simulink model "shape_delay_atten_noComp"  (R2022a)
settings: Solver=FixedStepAuto  StartTime=0.0  StopTime=10.0  RelTol=1e-3
values from neighbouring files (symbols this model uses):
  f_atten = 0.1    [zz_noShape.m]
  scale_LED = a_LED(numel(a_LED)) * A0_stage^num_LED    [zz_noShape.m]
  scale_ZCD = a_ZCD(numel(a_ZCD)) * A0_stage^num_ZCD    [zz_noShape.m]
  t_delay = shaper_struct.t_delay;'    [sim_shaper.m]    (also in zz_cfd.m = 2e-9;'; zz_noShape.m = 1.337e-08)
  v_threshold = (1.8/(2^9)) * 71    (= 0.249609375)    [zz_noShape.m]
  voff_led = 0.0    (= 0)    [zz_noShape.m]
  voff_zcd = 0.0    (= 0)    [zz_noShape.m]
undefined symbols (not defined in the file or in its folder): a_LED, a_ZCD, b_LED, b_ZCD
settings Model: Creator=lydialee  LastModifiedBy=lydialee
settings SolverCC: MaxZcPerStep=1
settings DataIOCC: ExternalInput=[t_vec, v_in]

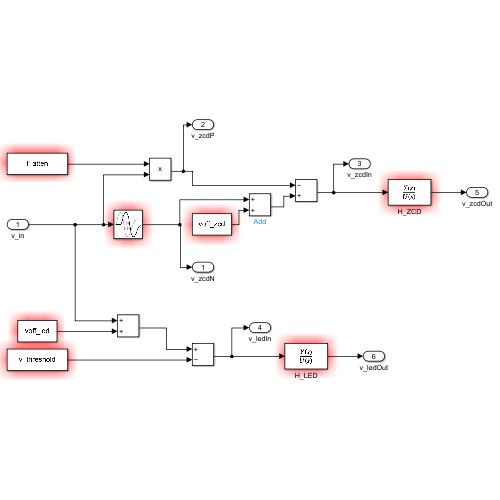
[thumbnail: Simulink's stored preview of the top-level diagram]
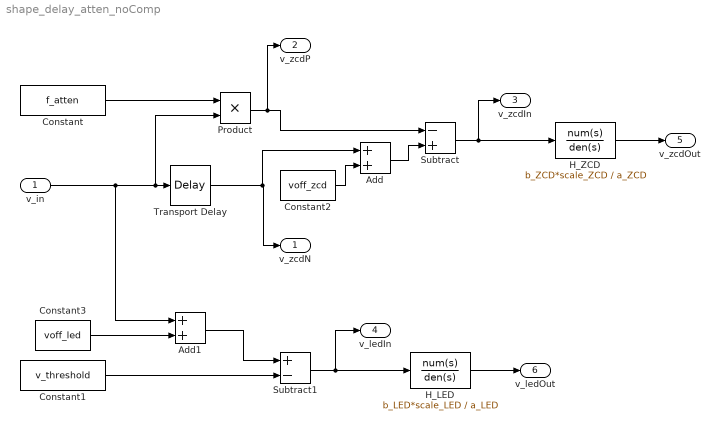
== system shape_delay_atten_noComp ==
  v_in : Inport
  Add : Sum
  Add1 : Sum
  Constant : Constant  Value=f_atten
  Constant1 : Constant  Value=v_threshold
  Constant2 : Constant  Value=voff_zcd
  Constant3 : Constant  Value=voff_led
  H_LED : TransferFcn  Numerator=b_LED*scale_LED  Denominator=a_LED
  H_ZCD : TransferFcn  Numerator=b_ZCD*scale_ZCD  Denominator=a_ZCD
  Product : Product
  Subtract : Sum  Inputs=-+
  Subtract1 : Sum  Inputs=+-
  Transport Delay : TransportDelay  DelayTime=t_delay
  v_zcdN : Outport  VectorParamsAs1DForOutWhenUnconnected=off
  v_zcdP : Outport  Port=2  VectorParamsAs1DForOutWhenUnconnected=off
  v_zcdIn : Outport  Port=3
  v_ledIn : Outport  Port=4
  v_zcdOut : Outport  Port=5
  v_ledOut : Outport  Port=6
  wires:
  Constant/1 -> Product/1
  v_in/1 -> Add1/1, Transport Delay/1, Product/2
  Transport Delay/1 -> Add/1, v_zcdN/1
  Product/1 -> v_zcdP/1, Subtract/1
  Constant1/1 -> Subtract1/2
  Subtract1/1 -> H_LED/1, v_ledIn/1
  Subtract/1 -> H_ZCD/1, v_zcdIn/1
  Add/1 -> Subtract/2
  Constant2/1 -> Add/2
  Add1/1 -> Subtract1/1
  Constant3/1 -> Add1/2
  H_LED/1 -> v_ledOut/1
  H_ZCD/1 -> v_zcdOut/1
